simulink library "spacar_lib"  (Simulink 3.00)
settings Model: Creator=AartsRGKM  LastModifiedBy=aarts

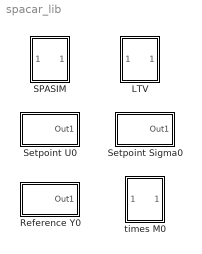
== system spacar_lib ==
  LTV : Subsystem  mask{filenm=, imode=Linear, nmodes=-1}
      mask prompts: filenm "SPACAR data filename"; imode "Interpolation type"; nmodes "Number of modes (-1 for all)"
      mask init:
      | if size(who('filenm'))>0; dfilenm=filenm; else; dfilenm=''; end; if nmodes>0; dfilenm=[ dfilenm '\n(' num2str(nmodes) ' modes)']; end;
      mask StyleString: edit,popup(Stepwise|Linear),edit
      mask Display: disp(dfilenm);
  Reference Y0 : Subsystem  mask{filenm=, imode=Spline}
      mask prompts: filenm "SPACAR data filename"; imode "Interpolation type"
      mask init:
      | if size(who('filenm'))>0; dfilenm=filenm; else; dfilenm=''; end
      mask StyleString: edit,popup(Stepwise|Linear|Spline)
      mask Display: disp(dfilenm);
  SPASIM : Subsystem  mask{filenm=, plot=off, sbdout=off}
      mask prompts: filenm "SPACAR data filename"; plot "Open graphical window"; sbdout "Write SBD file"
      mask init:
      | if size(who('filenm'))>0; dfilenm=filenm; else; dfilenm=''; end
      mask Display: disp(dfilenm);
  Setpoint Sigma0 : Subsystem  mask{filenm=, imode=Spline}
      mask prompts: filenm "SPACAR data filename"; imode "Interpolation type"
      mask init:
      | if size(who('filenm'))>0; dfilenm=filenm; else; dfilenm=''; end
      mask StyleString: edit,popup(Stepwise|Linear|Spline)
      mask Display: disp(dfilenm);
  Setpoint U0 : Subsystem  mask{filenm=, imode=Spline}
      mask prompts: filenm "SPACAR data filename"; imode "Interpolation type"
      mask init:
      | if size(who('filenm'))>0; dfilenm=filenm; else; dfilenm=''; end
      mask StyleString: edit,popup(Stepwise|Linear|Spline)
      mask Display: disp(dfilenm);
  times M0 : Subsystem  mask{filenm=, imode=Spline, nmodes=-1}
      mask prompts: filenm "SPACAR data filename"; imode "Interpolation type"; nmodes "Number of modes (-1 for all)"
      mask init:
      | if size(who('filenm'))>0; dfilenm=filenm; else; dfilenm=''; end; if nmodes>0; dfilenm=[ dfilenm '\n(' num2str(nmodes) ' modes)']; end;
      mask StyleString: edit,popup(Stepwise|Linear|Spline),edit
      mask Display: disp(dfilenm);

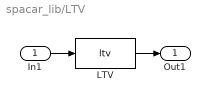
== system spacar_lib/LTV ==
  In1 : Inport  Port=1  PortWidth=-1  SampleTime=-1  DataType=auto
      settings: SignalType=auto
  LTV : S-Function  FunctionName=ltv  Parameters="filenm, [  0 imode-1 nmodes]"  PortCounts=[]  SFunctionModules=''
  Out1 : Outport  Port=1  InitialOutput=0
  wires:
  LTV/1 -> Out1/1
  In1/1 -> LTV/1

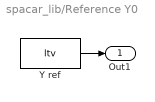
== system spacar_lib/Reference Y0 ==
  Y ref : S-Function  FunctionName=ltv  Parameters=filenm, [12 imode-1]  PortCounts=[]  SFunctionModules=''
  Out1 : Outport  Port=1  InitialOutput=0
  wires:
  Y ref/1 -> Out1/1

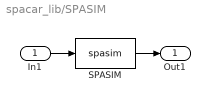
== system spacar_lib/SPASIM ==
  In1 : Inport  Port=1  PortWidth=-1  SampleTime=-1  DataType=auto
      settings: SignalType=auto
  SPASIM : S-Function  FunctionName=spasim  Parameters=filenm,plot,sbdout  PortCounts=[]  SFunctionModules=''
  Out1 : Outport  Port=1  InitialOutput=0
  wires:
  In1/1 -> SPASIM/1
  SPASIM/1 -> Out1/1

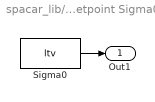
== system spacar_lib/Setpoint Sigma0 ==
  Sigma0 : S-Function  FunctionName=ltv  Parameters=filenm, [ 13 imode-1]  PortCounts=[]  SFunctionModules=''
  Out1 : Outport  Port=1  InitialOutput=0
  wires:
  Sigma0/1 -> Out1/1

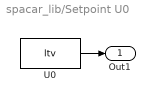
== system spacar_lib/Setpoint U0 ==
  U0 : S-Function  FunctionName=ltv  Parameters=filenm, [ 11 imode-1]  PortCounts=[]  SFunctionModules=''
  Out1 : Outport  Port=1  InitialOutput=0
  wires:
  U0/1 -> Out1/1

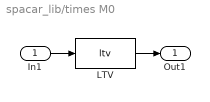
== system spacar_lib/times M0 ==
  In1 : Inport  Port=1  PortWidth=-1  SampleTime=-1  DataType=auto
      settings: SignalType=auto
  LTV : S-Function  FunctionName=ltv  Parameters="filenm, [  31 imode-1 nmodes]"  PortCounts=[]  SFunctionModules=''
  Out1 : Outport  Port=1  InitialOutput=0
  wires:
  In1/1 -> LTV/1
  LTV/1 -> Out1/1
